simulink model "main"  (R2022a)
settings: Solver=FixedStepDiscrete  StartTime=0.0  StopTime=Inf  FixedStep=(50e-6)-(sim_en*4.995e-5)  RelTol=1e-3  EnableMultiTasking=on
model workspace (MAT data in the model file):
  Param : Simulink.Parameter (value not decoded)
  ac_ok : Simulink.Signal (value not decoded)
  ac_ok_120 : Simulink.Signal (value not decoded)
  bulk_voltage : Simulink.Signal (value not decoded)
  burstduty_integ_max : Simulink.Signal (value not decoded)
  burstduty_integ_min : Simulink.Signal (value not decoded)
  burstduty_ki : Simulink.Signal (value not decoded)
  burstduty_kp : Simulink.Signal (value not decoded)
  calib_ok : Simulink.Signal (value not decoded)
  can_addr1 : Simulink.Signal (value not decoded)
  can_addr2 : Simulink.Signal (value not decoded)
  can_addr3 : Simulink.Signal (value not decoded)
  can_addr4 : Simulink.Signal (value not decoded)
  can_data_rx : Simulink.Signal (value not decoded)
  can_data_tx : Simulink.Signal (value not decoded)
  can_timeout_120 : Simulink.Signal (value not decoded)
  chksum_scircv : Simulink.Signal (value not decoded)
  clllc_en_120 : Simulink.Signal (value not decoded)
  clllc_fault_120 : Simulink.Signal (value not decoded)
  clllc_ok_120 : Simulink.Signal (value not decoded)
  cmpss1h : Simulink.Signal (value not decoded)
  cmpss1l : Simulink.Signal (value not decoded)
  cmpss2h : Simulink.Signal (value not decoded)
  cmpss2l : Simulink.Signal (value not decoded)
  cmpss3h : Simulink.Signal (value not decoded)
  cmpss3l : Simulink.Signal (value not decoded)
  cmpss4h : Simulink.Signal (value not decoded)
  cmpss4l : Simulink.Signal (value not decoded)
  cmpss5h : Simulink.Signal (value not decoded)
  cmpss5l : Simulink.Signal (value not decoded)
  cmpss6h : Simulink.Signal (value not decoded)
  cmpss6l : Simulink.Signal (value not decoded)
  cmpss7h : Simulink.Signal (value not decoded)
  cmpss7l : Simulink.Signal (value not decoded)
  cmpss8h : Simulink.Signal (value not decoded)
  cmpss8l : Simulink.Signal (value not decoded)
  cnt_idle : Simulink.Signal (value not decoded)
  cnt_orps : Simulink.Signal (value not decoded)
  cnt_scircv : Simulink.Signal (value not decoded)
  cnt_scixmt : Simulink.Signal (value not decoded)
  cnt_scixmt_func : Simulink.Signal (value not decoded)
  cnt_temp_mux : Simulink.Signal (value not decoded)
  cnt_vdroop : Simulink.Signal (value not decoded)
  config_ok : Simulink.Signal (value not decoded)
  control_en : Simulink.Signal (value not decoded)
  cp_ready_120 : Simulink.Signal (value not decoded)
  d2d_en : Simulink.Signal (value not decoded)
  dchg_off : Simulink.Signal (value not decoded)
  debug_dacb : Simulink.Signal (value not decoded)
  debug_dacc : Simulink.Signal (value not decoded)
  debug_msg1 : Simulink.Signal (value not decoded)
  debug_msg2 : Simulink.Signal (value not decoded)
  debug_msg3 : Simulink.Signal (value not decoded)
  debug_msg4 : Simulink.Signal (value not decoded)
  debug_msg5 : Simulink.Signal (value not decoded)
  debug_msg6 : Simulink.Signal (value not decoded)
  dir_v2g : Simulink.Signal (value not decoded)
  eoss_llc1 : Simulink.Signal (value not decoded)
  eoss_llc2 : Simulink.Signal (value not decoded)
  eoss_orps : Simulink.Signal (value not decoded)
  fault_ocp : Simulink.Signal (value not decoded)
  fault_otp : Simulink.Signal (value not decoded)
  fault_ovp : Simulink.Signal (value not decoded)
  fut_en : Simulink.Signal (value not decoded)
  fwd_en_120 : Simulink.Signal (value not decoded)
  gain_llc1_sec_idc : Simulink.Signal (value not decoded)
  gain_llc1_temp_sr : Simulink.Signal (value not decoded)
  gain_llc2_sec_idc : Simulink.Signal (value not decoded)
  gain_vbat : Simulink.Signal (value not decoded)
  gain_vbulk : Simulink.Signal (value not decoded)
  gain_vout : Simulink.Signal (value not decoded)
  input_current_phasea : Simulink.Signal (value not decoded)
  input_current_phaseb : Simulink.Signal (value not decoded)
  input_current_phasec : Simulink.Signal (value not decoded)
  input_freq : Simulink.Signal (value not decoded)
  input_power : Simulink.Signal (value not decoded)
  input_voltage_phasea : Simulink.Signal (value not decoded)
  input_voltage_phaseb : Simulink.Signal (value not decoded)
  input_voltage_phasec : Simulink.Signal (value not decoded)
  ishare_arbiter : Simulink.Signal (value not decoded)
  ishare_thresh : Simulink.Signal (value not decoded)
  led_g : Simulink.Signal (value not decoded)
  led_r : Simulink.Signal (value not decoded)
  led_y : Simulink.Signal (value not decoded)
  llc1_burst_integ : Simulink.Signal (value not decoded)
  llc1_burstduty_buffer : Simulink.Signal (value not decoded)
  llc1_pfm_error : Simulink.Signal (value not decoded)
  llc1_pfm_integ : Simulink.Signal (value not decoded)
  llc1_pfm_prop : Simulink.Signal (value not decoded)
  llc1_pri_idc : Simulink.Signal (value not decoded)
  llc1_ps_buffer : Simulink.Signal (value not decoded)
  llc1_pspwm_error : Simulink.Signal (value not decoded)
  llc1_pspwm_integ : Simulink.Signal (value not decoded)
  llc1_pspwm_prop : Simulink.Signal (value not decoded)
  llc1_sec_idc : Simulink.Signal (value not decoded)
  llc1_temp_sr : Simulink.Signal (value not decoded)
  llc1_ts_tbctr_buffer : Simulink.Signal (value not decoded)
  llc2_burst_integ : Simulink.Signal (value not decoded)
  llc2_burstduty_buffer : Simulink.Signal (value not decoded)
  llc2_en : Simulink.Signal (value not decoded)
  llc2_en_buffer : Simulink.Signal (value not decoded)
  llc2_pfm_error : Simulink.Signal (value not decoded)
  llc2_pfm_integ : Simulink.Signal (value not decoded)
  llc2_pfm_prop : Simulink.Signal (value not decoded)
  llc2_pri_idc : Simulink.Signal (value not decoded)
  llc2_ps_buffer : Simulink.Signal (value not decoded)
  llc2_pspwm_error : Simulink.Signal (value not decoded)
  llc2_pspwm_integ : Simulink.Signal (value not decoded)
  llc2_pspwm_prop : Simulink.Signal (value not decoded)
  llc2_sec_idc : Simulink.Signal (value not decoded)
  llc2_temp_sr : Simulink.Signal (value not decoded)
  llc2_ts_tbctr_buffer : Simulink.Signal (value not decoded)
  loop_adcint : Simulink.Signal (value not decoded)
  loop_control : Simulink.Signal (value not decoded)
  loop_idle : Simulink.Signal (value not decoded)
  mid_bulk_voltage : Simulink.Signal (value not decoded)
  mode_120 : Simulink.Signal (value not decoded)
  mode_cc_cv : Simulink.Signal (value not decoded)
  myParam : mpt.Parameter (value not decoded)
  obc_ok_120 : Simulink.Signal (value not decoded)
  offset_llc1_sec_idc : Simulink.Signal (value not decoded)
  offset_llc1_temp_sr : Simulink.Signal (value not decoded)
  offset_llc2_sec_idc : Simulink.Signal (value not decoded)
  offset_vbat : Simulink.Signal (value not decoded)
  offset_vbulk : Simulink.Signal (value not decoded)
  offset_vout : Simulink.Signal (value not decoded)
  openloop_en : Simulink.Signal (value not decoded)
  openloop_fault_en : Simulink.Signal (value not decoded)
  ot_fault_120 : Simulink.Signal (value not decoded)
  pfc_en : Simulink.Signal (value not decoded)
  pfc_en_120 : Simulink.Signal (value not decoded)
  pfc_fw_revision : Simulink.Signal (value not decoded)
  pfc_fw_revision_bootloader : Simulink.Signal (value not decoded)
  pfc_fw_revision_debug : Simulink.Signal (value not decoded)
  pfc_ok : Simulink.Signal (value not decoded)
  pfc_ok_120 : Simulink.Signal (value not decoded)
  pfm_a0 : Simulink.Signal (value not decoded)
  pfm_a1 : Simulink.Signal (value not decoded)
  pfm_integ_max : Simulink.Signal (value not decoded)
  pfm_integ_min : Simulink.Signal (value not decoded)
  pfm_ki : Simulink.Signal (value not decoded)
  pfm_kp : Simulink.Signal (value not decoded)
  pri_fut_en : Simulink.Signal (value not decoded)
  pri_fut_en_buffer : Simulink.Signal (value not decoded)
  pri_halfbridge_en : Simulink.Signal (value not decoded)
  pri_halfbridge_en_buffer : Simulink.Signal (value not decoded)
  pspwm_integ_max : Simulink.Signal (value not decoded)
  pspwm_integ_min : Simulink.Signal (value not decoded)
  pspwm_ki : Simulink.Signal (value not decoded)
  pspwm_kp : Simulink.Signal (value not decoded)
  ref_idclink_max : Simulink.Signal (value not decoded)
  ref_iout : Simulink.Signal (value not decoded)
  ref_iout_calib : Simulink.Signal (value not decoded)
  ref_iout_llc1 : Simulink.Signal (value not decoded)
  ref_iout_llc1_calib : Simulink.Signal (value not decoded)
  ref_iout_llc2 : Simulink.Signal (value not decoded)
  ref_iout_llc2_calib : Simulink.Signal (value not decoded)
  ref_pout : Simulink.Signal (value not decoded)
  ref_ss_llc1 : Simulink.Signal (value not decoded)
  ref_ss_llc2 : Simulink.Signal (value not decoded)
  ref_ss_orps : Simulink.Signal (value not decoded)
  ref_vbat : Simulink.Signal (value not decoded)
  ref_vbat_calib : Simulink.Signal (value not decoded)
  ref_vbulk : Simulink.Signal (value not decoded)
  ref_vbulk_calib : Simulink.Signal (value not decoded)
  ref_vbulk_llc1_calib : Simulink.Signal (value not decoded)
  ref_vbulk_llc2_calib : Simulink.Signal (value not decoded)
  ref_vout : Simulink.Signal (value not decoded)
  ref_vout_calib : Simulink.Signal (value not decoded)
  relay_en : Simulink.Signal (value not decoded)
  reset_flag : Simulink.Signal (value not decoded)
  rev_en_120 : Simulink.Signal (value not decoded)
  runtime_control : Simulink.Signal (value not decoded)
  runtime_idle : Simulink.Signal (value not decoded)
  scircv_buffer : Simulink.Signal (value not decoded)
  scircv_buffer_tmp : Simulink.Signal (value not decoded)
  scircv_buffer_tmp_idx0 : Simulink.Signal (value not decoded)
  scircv_chksum : Simulink.Signal (value not decoded)
  scircv_chksum_ok : Simulink.Signal (value not decoded)
  scircv_parse_ok : Simulink.Signal (value not decoded)
  scixmt_buffer : Simulink.Signal (value not decoded)
  scixmt_chksum : Simulink.Signal (value not decoded)
  scixmt_func : Simulink.Signal (value not decoded)
  scixmt_word0_lsb : Simulink.Signal (value not decoded)
  scixmt_word0_msb : Simulink.Signal (value not decoded)
  scixmt_word1_lsb : Simulink.Signal (value not decoded)
  scixmt_word1_msb : Simulink.Signal (value not decoded)
  scixmt_word2_lsb : Simulink.Signal (value not decoded)
  scixmt_word2_msb : Simulink.Signal (value not decoded)
  scixmt_wr : Simulink.Signal (value not decoded)
  ss_step : Simulink.Signal (value not decoded)
  state_calib : Simulink.Signal (value not decoded)
  state_control : Simulink.Signal (value not decoded)
  state_hkeep : Simulink.Signal (value not decoded)
  status_cmpss : Simulink.Signal (value not decoded)
  status_control : Simulink.Signal (value not decoded)
  status_digin : Simulink.Signal (value not decoded)
  status_digout : Simulink.Signal (value not decoded)
  status_fault : Simulink.Signal (value not decoded)
  status_input : Simulink.Signal (value not decoded)
  status_pfc : Simulink.Signal (value not decoded)
  temp_inlet : Simulink.Signal (value not decoded)
  temp_llc1_fet_hs : Simulink.Signal (value not decoded)
  temp_llc2_fet_hs : Simulink.Signal (value not decoded)
  temp_mux : Simulink.Signal (value not decoded)
  temp_mux_s0 : Simulink.Signal (value not decoded)
  temp_mux_s1 : Simulink.Signal (value not decoded)
  temp_mux_s2 : Simulink.Signal (value not decoded)
  temp_outlet : Simulink.Signal (value not decoded)
  temp_pfc_fet_hsa : Simulink.Signal (value not decoded)
  temp_pfc_fet_hsb : Simulink.Signal (value not decoded)
  temp_pfc_fet_hsc : Simulink.Signal (value not decoded)
  temp_pfc_fet_lsa : Simulink.Signal (value not decoded)
  temp_pfc_fet_lsb : Simulink.Signal (value not decoded)
  temp_pfc_fet_lsc : Simulink.Signal (value not decoded)
  test_mode : Simulink.Signal (value not decoded)
  tfcv_cc : Simulink.Signal (value not decoded)
  tfcv_cc_llc2 : Simulink.Signal (value not decoded)
  tfcv_cv : Simulink.Signal (value not decoded)
  tfcv_sr_en : Simulink.Signal (value not decoded)
  tfv_assert_llc1_pri_idc : Simulink.Signal (value not decoded)
  tfv_assert_llc1_sec_idc : Simulink.Signal (value not decoded)
  tfv_assert_llc1_temp_sr : Simulink.Signal (value not decoded)
  tfv_assert_llc2_pri_idc : Simulink.Signal (value not decoded)
  tfv_assert_llc2_sec_idc : Simulink.Signal (value not decoded)
  tfv_assert_llc2_temp_sr : Simulink.Signal (value not decoded)
  tfv_assert_temp_outlet : Simulink.Signal (value not decoded)
  tfv_assert_vaux_uv : Simulink.Signal (value not decoded)
  tfv_assert_vbat : Simulink.Signal (value not decoded)
  tfv_assert_vbulk : Simulink.Signal (value not decoded)
  tfv_assert_vout : Simulink.Signal (value not decoded)
  tfv_cnt_tz : Simulink.Signal (value not decoded)
  tfv_deassert_llc1_pri_idc : Simulink.Signal (value not decoded)
  tfv_deassert_llc1_sec_idc : Simulink.Signal (value not decoded)
  tfv_deassert_llc1_temp_sr : Simulink.Signal (value not decoded)
  tfv_deassert_llc2_pri_idc : Simulink.Signal (value not decoded)
  tfv_deassert_llc2_sec_idc : Simulink.Signal (value not decoded)
  tfv_deassert_llc2_temp_sr : Simulink.Signal (value not decoded)
  tfv_deassert_temp_outlet : Simulink.Signal (value not decoded)
  tfv_deassert_vaux_uv : Simulink.Signal (value not decoded)
  tfv_deassert_vbat : Simulink.Signal (value not decoded)
  tfv_deassert_vbulk : Simulink.Signal (value not decoded)
  tfv_deassert_vout : Simulink.Signal (value not decoded)
  tfv_llc1_pri_idc : Simulink.Signal (value not decoded)
  tfv_llc1_sec_idc : Simulink.Signal (value not decoded)
  tfv_llc1_temp_sr : Simulink.Signal (value not decoded)
  tfv_llc2_pri_idc : Simulink.Signal (value not decoded)
  tfv_llc2_sec_idc : Simulink.Signal (value not decoded)
  tfv_llc2_temp_sr : Simulink.Signal (value not decoded)
  tfv_temp_outlet : Simulink.Signal (value not decoded)
  tfv_vaux_uv : Simulink.Signal (value not decoded)
  tfv_vbat : Simulink.Signal (value not decoded)
  tfv_vbulk : Simulink.Signal (value not decoded)
  tfv_vout : Simulink.Signal (value not decoded)
  timer_1ms : Simulink.Signal (value not decoded)
  tz : Simulink.Signal (value not decoded)
  valve_en : Simulink.Signal (value not decoded)
  vaux : Simulink.Signal (value not decoded)
  vbat : Simulink.Signal (value not decoded)
  vbulk : Simulink.Signal (value not decoded)
  vout : Simulink.Signal (value not decoded)
undefined symbols (not defined in the file or in its folder): CAN_O_INT, CANA_BASE, Down, GPTRIP1SEL, GPTRIP2SEL, TZ1, TZ2, Up
libraries: hdlsllib x159, simulink x100, c2837xDlib x24, c2807xlib x16, c280xlib x13, c2802xlib x12, canmsglib x8, idelinklib_common x2, c2000lib x1, c281xlib x1
(part 12 of 15)

== system main/Task_Manager/idle/idle_task/status/init/digin//digout_variant_subsystem/sim ==
  sim_digin : Inport
  Data Store Read : DataStoreRead  DataStoreName=dchg_off  IndexOptions=Index vector (dialog)  Indices=1  OutputSizes=1
  Data Store Read1 : DataStoreRead  DataStoreName=temp_mux_s0  IndexOptions=Index vector (dialog)  Indices=1  OutputSizes=1
  Data Store Read2 : DataStoreRead  DataStoreName=pfc_en  IndexOptions=Index vector (dialog)  Indices=1  OutputSizes=1
  Data Store Read3 : DataStoreRead  DataStoreName=temp_mux_s1  IndexOptions=Index vector (dialog)  Indices=1  OutputSizes=1
  Data Store Read4 : DataStoreRead  DataStoreName=temp_mux_s2  IndexOptions=Index vector (dialog)  Indices=1  OutputSizes=1
  Data Store Read5 : DataStoreRead  DataStoreName=valve_en  IndexOptions=Index vector (dialog)  Indices=1  OutputSizes=1
  Data Store Read6 : DataStoreRead  DataStoreName=relay_en  IndexOptions=Index vector (dialog)  Indices=1  OutputSizes=1
  Data Store Read7 : DataStoreRead  DataStoreName=led_r  IndexOptions=Index vector (dialog)  Indices=1  OutputSizes=1
  Data Store Read8 : DataStoreRead  DataStoreName=led_g  IndexOptions=Index vector (dialog)  Indices=1  OutputSizes=1
  Data Store Read9 : DataStoreRead  DataStoreName=led_y  IndexOptions=Index vector (dialog)  Indices=1  OutputSizes=1
  Data Store Write : DataStoreWrite  DataStoreName=ac_ok  IndexOptions=Index vector (dialog)  Indices=1  OutputSizes=1
  Data Store Write1 : DataStoreWrite  DataStoreName=can_addr1  IndexOptions=Index vector (dialog)  Indices=1  OutputSizes=1
  Data Store Write2 : DataStoreWrite  DataStoreName=can_addr2  IndexOptions=Index vector (dialog)  Indices=1  OutputSizes=1
  Data Store Write3 : DataStoreWrite  DataStoreName=can_addr3  IndexOptions=Index vector (dialog)  Indices=1  OutputSizes=1
  Data Store Write4 : DataStoreWrite  DataStoreName=can_addr4  IndexOptions=Index vector (dialog)  Indices=1  OutputSizes=1
  Data Store Write5 : DataStoreWrite  DataStoreName=pfc_ok  IndexOptions=Index vector (dialog)  Indices=1  OutputSizes=1
  Demux : Demux  Outputs=7
  Mux : Mux  Inputs=10
  sim_digout : Outport
  wires:
  sim_digin/1 -> Demux/1
  Demux/6 -> Data Store Write/1
  Demux/7 -> ?
  Demux/1 -> Data Store Write1/1
  Demux/2 -> Data Store Write2/1
  Demux/3 -> Data Store Write3/1
  Demux/4 -> Data Store Write4/1
  Demux/5 -> Data Store Write5/1
  Mux/1 -> sim_digout/1
  Data Store Read7/1 -> Mux/1
  Data Store Read8/1 -> Mux/2
  Data Store Read5/1 -> Mux/9
  Data Store Read4/1 -> Mux/8
  Data Store Read3/1 -> Mux/7
  Data Store Read1/1 -> Mux/6
  Data Store Read/1 -> Mux/4
  Data Store Read2/1 -> Mux/5
  Data Store Read9/1 -> Mux/3
  Data Store Read6/1 -> Mux/10

== system main/Task_Manager/idle/idle_task/status/update_CAN_msg1/OBC_CTRL_MSG_100/G2V_Forward_ON_A2 ==
  Action Port : ActionPort  ActionPortLabel=case [ 162 ]:
  Constant : Constant  Value=0  OutDataTypeStr=boolean  SampleTime=-1
  Constant1 : Constant  OutDataTypeStr=boolean  SampleTime=-1
  Data Store Write1 : DataStoreWrite  DataStoreName=fwd_en_120  IndexOptions=Index vector (dialog)  Indices=1  OutputSizes=1
  Data Store Write16 : DataStoreWrite  DataStoreName=dir_v2g  IndexOptions=Index vector (dialog)  Indices=1  OutputSizes=1
  wires:
  Constant/1 -> Data Store Write16/1
  Constant1/1 -> Data Store Write1/1

== system main/Task_Manager/idle/idle_task/status/update_CAN_msg1/OBC_CTRL_MSG_100/Sleep_A0 ==
  Action Port : ActionPort  ActionPortLabel=case [ 160 ]:
  Constant : Constant  Value=0  OutDataTypeStr=boolean
  Data Store Write16 : DataStoreWrite  DataStoreName=control_en  IndexOptions=Index vector (dialog)  Indices=1  OutputSizes=1
  wires:
  Constant/1 -> Data Store Write16/1

== system main/Task_Manager/idle/idle_task/status/update_CAN_msg1/OBC_CTRL_MSG_100/Stand-by_A1 ==
  Action Port : ActionPort  ActionPortLabel=case [ 161 ]:
  Constant : Constant  OutDataTypeStr=boolean
  Constant2 : Constant  Value=0  OutDataTypeStr=boolean  SampleTime=-1
  Data Store Write1 : DataStoreWrite  DataStoreName=rev_en_120  IndexOptions=Index vector (dialog)  Indices=1  OutputSizes=1
  Data Store Write16 : DataStoreWrite  DataStoreName=control_en  IndexOptions=Index vector (dialog)  Indices=1  OutputSizes=1
  Data Store Write2 : DataStoreWrite  DataStoreName=fwd_en_120  IndexOptions=Index vector (dialog)  Indices=1  OutputSizes=1
  wires:
  Constant/1 -> Data Store Write16/1
  Constant2/1 -> Data Store Write1/1, Data Store Write2/1

== system main/Task_Manager/idle/idle_task/status/update_CAN_msg1/OBC_CTRL_MSG_100/Test_mode_ON_AND_FWD_A4 ==
  Action Port : ActionPort  ActionPortLabel=case [ 164 ]:
  Constant : Constant  OutDataTypeStr=boolean
  Constant1 : Constant  Value=0  OutDataTypeStr=boolean  SampleTime=-1
  Data Store Write1 : DataStoreWrite  DataStoreName=dir_v2g  IndexOptions=Index vector (dialog)  Indices=1  OutputSizes=1
  Data Store Write16 : DataStoreWrite  DataStoreName=test_mode  IndexOptions=Index vector (dialog)  Indices=1  OutputSizes=1
  wires:
  Constant/1 -> Data Store Write16/1
  Constant1/1 -> Data Store Write1/1

== system main/Task_Manager/idle/idle_task/status/update_CAN_msg1/OBC_CTRL_MSG_100/Test_mode_ON_AND_REV_A5 ==
  Action Port : ActionPort  ActionPortLabel=case [ 165 ]:
  Constant : Constant  OutDataTypeStr=boolean
  Constant1 : Constant  OutDataTypeStr=boolean  SampleTime=-1
  Data Store Write1 : DataStoreWrite  DataStoreName=dir_v2g  IndexOptions=Index vector (dialog)  Indices=1  OutputSizes=1
  Data Store Write16 : DataStoreWrite  DataStoreName=test_mode  IndexOptions=Index vector (dialog)  Indices=1  OutputSizes=1
  wires:
  Constant/1 -> Data Store Write16/1
  Constant1/1 -> Data Store Write1/1

== system main/Task_Manager/idle/idle_task/status/update_CAN_msg1/OBC_CTRL_MSG_100/V2G_Reverse_ON_A3 ==
  Action Port : ActionPort  ActionPortLabel=case [ 163 ]:
  Constant : Constant  OutDataTypeStr=boolean
  Constant2 : Constant  OutDataTypeStr=boolean  SampleTime=-1
  Data Store Write16 : DataStoreWrite  DataStoreName=dir_v2g  IndexOptions=Index vector (dialog)  Indices=1  OutputSizes=1
  Data Store Write2 : DataStoreWrite  DataStoreName=rev_en_120  IndexOptions=Index vector (dialog)  Indices=1  OutputSizes=1
  wires:
  Constant/1 -> Data Store Write16/1
  Constant2/1 -> Data Store Write2/1

== system main/Task_Manager/idle/idle_task/status/update_CAN_msg1/OBC_SEC_DATA2_141/Subsystem3 ==
  adc : Inport
  zero_offset : Inport  Port=2
  gain : Inport  Port=3
  Abs : Abs  SaturateOnIntegerOverflow=off
  Product6 : Product  OutDataTypeStr=single
  Saturation1 : Saturate  UpperLimit=4095  LowerLimit=0  OutDataTypeStr=single
  Subtract : Sum  Inputs=+-  AccumDataTypeStr=single  OutDataTypeStr=single
  actual : Outport
  wires:
  Product6/1 -> actual/1
  gain/1 -> Product6/2
  adc/1 -> Subtract/1
  zero_offset/1 -> Subtract/2
  Subtract/1 -> Abs/1
  Saturation1/1 -> Product6/1
  Abs/1 -> Saturation1/1

== system main/Task_Manager/idle/idle_task/status/update_CAN_msg1/OBC_SEC_DATA4_143/Subsystem ==
  Add : Sum  Inputs=++++++++
  Bit Shift1 : hdlsllib/Logic and Bit Operations/Bit Shift  mode=Shift Left Logical  N=1
  Bit Shift2 : hdlsllib/Logic and Bit Operations/Bit Shift  mode=Shift Left Logical  N=2
  Bit Shift3 : hdlsllib/Logic and Bit Operations/Bit Shift  mode=Shift Left Logical  N=3
  Bit Shift4 : hdlsllib/Logic and Bit Operations/Bit Shift  mode=Shift Left Logical  N=5
  Bit Shift5 : hdlsllib/Logic and Bit Operations/Bit Shift  mode=Shift Left Logical  N=6
  Bit Shift6 : hdlsllib/Logic and Bit Operations/Bit Shift  mode=Shift Left Logical  N=4
  Bit Shift7 : hdlsllib/Logic and Bit Operations/Bit Shift  mode=Shift Left Logical  N=7
  Data Store Read10 : DataStoreRead  DataStoreName=dir_v2g  IndexOptions=Index vector (dialog)  Indices=1  OutputSizes=1
  Data Store Read11 : DataStoreRead  DataStoreName=eoss_llc1  IndexOptions=Index vector (dialog)  Indices=1  OutputSizes=1
  Data Store Read12 : DataStoreRead  DataStoreName=calib_ok  IndexOptions=Index vector (dialog)  Indices=1  OutputSizes=1
  Data Store Read13 : DataStoreRead  DataStoreName=openloop_en  IndexOptions=Index vector (dialog)  Indices=1  OutputSizes=1
  Data Store Read14 : DataStoreRead  DataStoreName=fut_en  IndexOptions=Index vector (dialog)  Indices=1  OutputSizes=1
  Data Store Read4 : DataStoreRead  DataStoreName=eoss_llc2  IndexOptions=Index vector (dialog)  Indices=1  OutputSizes=1
  Data Store Read7 : DataStoreRead  DataStoreName=config_ok  IndexOptions=Index vector (dialog)  Indices=1  OutputSizes=1
  Data Store Read9 : DataStoreRead  DataStoreName=control_mode  IndexOptions=Index vector (dialog)  Indices=1  OutputSizes=1
  Data Store Write1 : DataStoreWrite  DataStoreName=sSecCtrlState  IndexOptions=Index vector (dialog)  Indices=1  OutputSizes=1
  Data Store Memory : DataStoreMemory  DataStoreName=control_mode  WriteAfterWriteMsg=warning  ShowAdditionalParam=off
  Data Type Conversion{,1..7,11} (9 alike) : DataTypeConversion  OutDataTypeStr=uint8  SaturateOnIntegerOverflow=off  RndMeth=Floor
  wires:
  Data Store Read11/1 -> Data Type Conversion4/1
  Bit Shift7/1 -> Add/8
  Data Type Conversion7/1 -> Bit Shift7/1
  Data Store Read9/1 -> Data Type Conversion/1
  Data Type Conversion2/1 -> Bit Shift2/1
  Bit Shift1/1 -> Add/2
  Bit Shift5/1 -> Add/7
  Data Store Read14/1 -> Data Type Conversion6/1
  Data Type Conversion5/1 -> Bit Shift4/1
  Bit Shift6/1 -> Add/5
  Data Type Conversion11/1 -> Data Store Write1/1
  Data Store Read13/1 -> Data Type Conversion7/1
  Data Type Conversion4/1 -> Bit Shift6/1
  Data Store Read4/1 -> Data Type Conversion5/1
  Data Store Read10/1 -> Data Type Conversion1/1
  Data Type Conversion/1 -> Add/1
  Bit Shift2/1 -> Add/3
  Bit Shift4/1 -> Add/6
  Add/1 -> Data Type Conversion11/1
  Data Type Conversion1/1 -> Bit Shift1/1
  Data Store Read7/1 -> Data Type Conversion3/1
  Data Store Read12/1 -> Data Type Conversion2/1
  Data Type Conversion6/1 -> Bit Shift5/1
  Data Type Conversion3/1 -> Bit Shift3/1
  Bit Shift3/1 -> Add/4

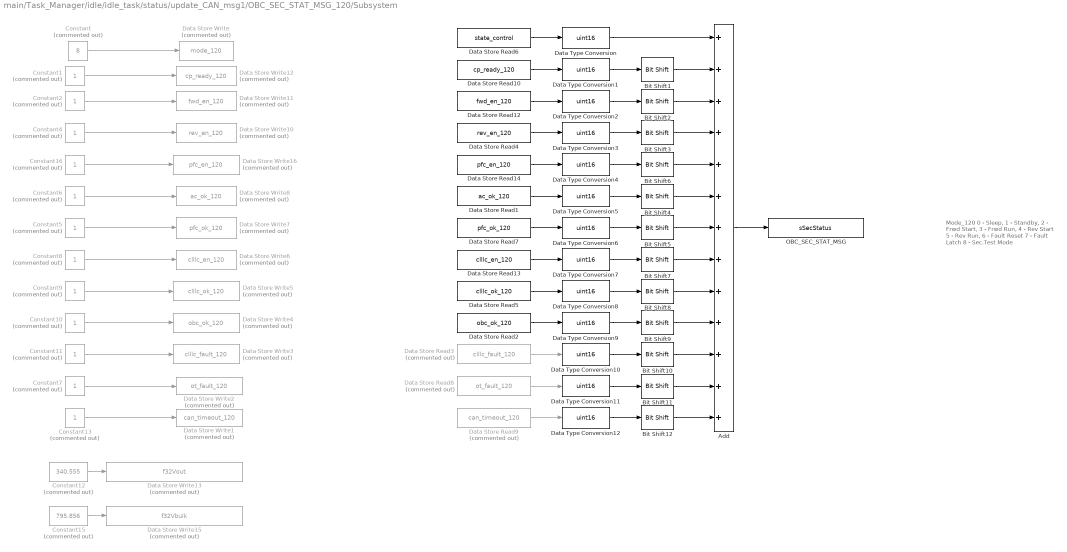
== system main/Task_Manager/idle/idle_task/status/update_CAN_msg1/OBC_SEC_STAT_MSG_120/Subsystem ==
  note: Mode_120
      |
      | 0 - Sleep,
      | 1 - Standby,
      | 2 - Frwd Start,
      | 3 - Frwd Run,
      | 4 - Rev Start
      | 5 - Rev Run,
      | 6 - Fault Reset
      | 7 - Fault Latch
      | 8 - Sec.Test Mode
  Add : Sum  Inputs=+++++++++++++
  Bit Shift1 : hdlsllib/Logic and Bit Operations/Bit Shift  mode=Shift Left Logical  N=4
  Bit Shift10 : hdlsllib/Logic and Bit Operations/Bit Shift  mode=Shift Left Logical  N=13
  Bit Shift11 : hdlsllib/Logic and Bit Operations/Bit Shift  mode=Shift Left Logical  N=14
  Bit Shift12 : hdlsllib/Logic and Bit Operations/Bit Shift  mode=Shift Left Logical  N=15
  Bit Shift2 : hdlsllib/Logic and Bit Operations/Bit Shift  mode=Shift Left Logical  N=5
  Bit Shift3 : hdlsllib/Logic and Bit Operations/Bit Shift  mode=Shift Left Logical  N=6
  Bit Shift4 : hdlsllib/Logic and Bit Operations/Bit Shift  mode=Shift Left Logical  N=8
  Bit Shift5 : hdlsllib/Logic and Bit Operations/Bit Shift  mode=Shift Left Logical  N=9
  Bit Shift6 : hdlsllib/Logic and Bit Operations/Bit Shift  mode=Shift Left Logical  N=7
  Bit Shift7 : hdlsllib/Logic and Bit Operations/Bit Shift  mode=Shift Left Logical  N=10
  Bit Shift8 : hdlsllib/Logic and Bit Operations/Bit Shift  mode=Shift Left Logical  N=11
  Bit Shift9 : hdlsllib/Logic and Bit Operations/Bit Shift  mode=Shift Left Logical  N=12
  Constant : Constant  Commented=on  Value=8  OutDataTypeStr=uint8
  Constant{1..2,4..11,13,16} (12 alike) : Constant  Commented=on  OutDataTypeStr=boolean
  Constant12 : Constant  Commented=on  Value=340.555  OutDataTypeStr=single
  Constant15 : Constant  Commented=on  Value=795.856  OutDataTypeStr=single
  Data Store Read1 : DataStoreRead  DataStoreName=ac_ok_120  IndexOptions=Index vector (dialog)  Indices=1  OutputSizes=1
  Data Store Read10 : DataStoreRead  DataStoreName=cp_ready_120  IndexOptions=Index vector (dialog)  Indices=1  OutputSizes=1
  Data Store Read12 : DataStoreRead  DataStoreName=fwd_en_120  IndexOptions=Index vector (dialog)  Indices=1  OutputSizes=1
  Data Store Read13 : DataStoreRead  DataStoreName=clllc_en_120  IndexOptions=Index vector (dialog)  Indices=1  OutputSizes=1
  Data Store Read14 : DataStoreRead  DataStoreName=pfc_en_120  IndexOptions=Index vector (dialog)  Indices=1  OutputSizes=1
  Data Store Read2 : DataStoreRead  DataStoreName=obc_ok_120  IndexOptions=Index vector (dialog)  Indices=1  OutputSizes=1
  Data Store Read3 : DataStoreRead  Commented=on  DataStoreName=clllc_fault_120  IndexOptions=Index vector (dialog)  Indices=1  OutputSizes=1
  Data Store Read4 : DataStoreRead  DataStoreName=rev_en_120  IndexOptions=Index vector (dialog)  Indices=1  OutputSizes=1
  Data Store Read5 : DataStoreRead  DataStoreName=clllc_ok_120  IndexOptions=Index vector (dialog)  Indices=1  OutputSizes=1
  Data Store Read6 : DataStoreRead  DataStoreName=state_control  IndexOptions=Index vector (dialog)  Indices=1  OutputSizes=1
  Data Store Read7 : DataStoreRead  DataStoreName=pfc_ok_120  IndexOptions=Index vector (dialog)  Indices=1  OutputSizes=1
  Data Store Read8 : DataStoreRead  Commented=on  DataStoreName=ot_fault_120  IndexOptions=Index vector (dialog)  Indices=1  OutputSizes=1
  Data Store Read9 : DataStoreRead  Commented=on  DataStoreName=can_timeout_120  IndexOptions=Index vector (dialog)  Indices=1  OutputSizes=1
  Data Store Write : DataStoreWrite  Commented=on  DataStoreName=mode_120  IndexOptions=Index vector (dialog)  Indices=1  OutputSizes=1
  Data Store Write1 : DataStoreWrite  Commented=on  DataStoreName=can_timeout_120  IndexOptions=Index vector (dialog)  Indices=1  OutputSizes=1
  Data Store Write10 : DataStoreWrite  Commented=on  DataStoreName=rev_en_120  IndexOptions=Index vector (dialog)  Indices=1  OutputSizes=1
  Data Store Write11 : DataStoreWrite  Commented=on  DataStoreName=fwd_en_120  IndexOptions=Index vector (dialog)  Indices=1  OutputSizes=1
  Data Store Write12 : DataStoreWrite  Commented=on  DataStoreName=cp_ready_120  IndexOptions=Index vector (dialog)  Indices=1  OutputSizes=1
  Data Store Write13 : DataStoreWrite  Commented=on  DataStoreName=f32Vout  IndexOptions=Index vector (dialog)  Indices=1  OutputSizes=1
  Data Store Write15 : DataStoreWrite  Commented=on  DataStoreName=f32Vbulk  IndexOptions=Index vector (dialog)  Indices=1  OutputSizes=1
  Data Store Write16 : DataStoreWrite  Commented=on  DataStoreName=pfc_en_120  IndexOptions=Index vector (dialog)  Indices=1  OutputSizes=1
  Data Store Write2 : DataStoreWrite  Commented=on  DataStoreName=ot_fault_120  IndexOptions=Index vector (dialog)  Indices=1  OutputSizes=1
  Data Store Write3 : DataStoreWrite  Commented=on  DataStoreName=clllc_fault_120  IndexOptions=Index vector (dialog)  Indices=1  OutputSizes=1
  Data Store Write4 : DataStoreWrite  Commented=on  DataStoreName=obc_ok_120  IndexOptions=Index vector (dialog)  Indices=1  OutputSizes=1
  Data Store Write5 : DataStoreWrite  Commented=on  DataStoreName=clllc_ok_120  IndexOptions=Index vector (dialog)  Indices=1  OutputSizes=1
  Data Store Write6 : DataStoreWrite  Commented=on  DataStoreName=clllc_en_120  IndexOptions=Index vector (dialog)  Indices=1  OutputSizes=1
  Data Store Write7 : DataStoreWrite  Commented=on  DataStoreName=pfc_ok_120  IndexOptions=Index vector (dialog)  Indices=1  OutputSizes=1
  Data Store Write8 : DataStoreWrite  Commented=on  DataStoreName=ac_ok_120  IndexOptions=Index vector (dialog)  Indices=1  OutputSizes=1
  Data Type Conversion{,1..12} (13 alike) : DataTypeConversion  OutDataTypeStr=uint16  SaturateOnIntegerOverflow=off  RndMeth=Floor
  OBC_SEC_STAT_MSG : DataStoreWrite  DataStoreName=sSecStatus  IndexOptions=Index vector (dialog)  Indices=1  OutputSizes=1
  wires:
  Constant13/1 -> Data Store Write1/1
  Data Store Read12/1 -> Data Type Conversion2/1
  Data Type Conversion1/1 -> Bit Shift1/1
  Bit Shift3/1 -> Add/4
  Bit Shift1/1 -> Add/2
  Data Type Conversion4/1 -> Bit Shift6/1
  Data Type Conversion2/1 -> Bit Shift2/1
  Bit Shift2/1 -> Add/3
  Data Store Read1/1 -> Data Type Conversion5/1
  Bit Shift9/1 -> Add/10
  Data Type Conversion3/1 -> Bit Shift3/1
  Constant2/1 -> Data Store Write11/1
  Data Type Conversion10/1 -> Bit Shift10/1
  Data Store Read8/1 -> Data Type Conversion11/1
  Data Type Conversion7/1 -> Bit Shift7/1
  Data Store Read13/1 -> Data Type Conversion7/1
  Bit Shift8/1 -> Add/9
  Data Type Conversion8/1 -> Bit Shift8/1
  Data Store Read2/1 -> Data Type Conversion9/1
  Data Type Conversion6/1 -> Bit Shift5/1
  Bit Shift6/1 -> Add/5
  Constant5/1 -> Data Store Write7/1
  Constant1/1 -> Data Store Write12/1
  Data Store Read10/1 -> Data Type Conversion1/1
  Data Type Conversion9/1 -> Bit Shift9/1
  Data Type Conversion/1 -> Add/1
  Bit Shift4/1 -> Add/6
  Data Store Read4/1 -> Data Type Conversion3/1
  Bit Shift5/1 -> Add/7
  Constant/1 -> Data Store Write/1
  Data Store Read3/1 -> Data Type Conversion10/1
  Data Type Conversion5/1 -> Bit Shift4/1
  Data Store Read6/1 -> Data Type Conversion/1
  Data Store Read14/1 -> Data Type Conversion4/1
  Constant9/1 -> Data Store Write5/1
  Bit Shift11/1 -> Add/12
  Data Store Read5/1 -> Data Type Conversion8/1
  Bit Shift10/1 -> Add/11
  Data Store Read7/1 -> Data Type Conversion6/1
  Bit Shift7/1 -> Add/8
  Constant11/1 -> Data Store Write3/1
  Constant12/1 -> Data Store Write13/1
  Constant15/1 -> Data Store Write15/1
  Data Type Conversion12/1 -> Bit Shift12/1
  Bit Shift12/1 -> Add/13
  Add/1 -> OBC_SEC_STAT_MSG/1
  Constant8/1 -> Data Store Write6/1
  Constant7/1 -> Data Store Write2/1
  Constant10/1 -> Data Store Write4/1
  Data Type Conversion11/1 -> Bit Shift11/1
  Constant6/1 -> Data Store Write8/1
  Constant4/1 -> Data Store Write10/1
  Constant16/1 -> Data Store Write16/1
  Data Store Read9/1 -> Data Type Conversion12/1

== system main/Task_Manager/idle/idle_task/status/update_CAN_msg1/OBC_SEC_STAT_MSG_120/Subsystem3 ==
  adc : Inport
  zero_offset : Inport  Port=2
  gain : Inport  Port=3
  Abs : Abs  SaturateOnIntegerOverflow=off
  Product6 : Product  OutDataTypeStr=single
  Saturation1 : Saturate  UpperLimit=4095  LowerLimit=0  OutDataTypeStr=single
  Subtract : Sum  Inputs=+-  AccumDataTypeStr=single  OutDataTypeStr=single
  actual : Outport
  wires:
  Product6/1 -> actual/1
  gain/1 -> Product6/2
  adc/1 -> Subtract/1
  zero_offset/1 -> Subtract/2
  Subtract/1 -> Abs/1
  Saturation1/1 -> Product6/1
  Abs/1 -> Saturation1/1

== system main/Task_Manager/init/codegen/init/tztl_clb/clb/System Initialize ==

== system main/Task_Manager/init/codegen/init/tztl_clb/tzctl/System Initialize ==

== system main/Control_State_Machine/Control_Loop/control/configSr/configXbarEpwmtrip/codegen/g2v_prifullbridge/clb/System Outputs1 ==

== system main/Control_State_Machine/Control_Loop/control/configSr/configXbarEpwmtrip/codegen/g2v_prifullbridge/tzctl/System Outputs ==

== system main/Control_State_Machine/Control_Loop/control/configSr/configXbarEpwmtrip/codegen/v2g_prifullbridge/clb/System Outputs3 ==

== system main/Control_State_Machine/Control_Loop/control/configSr/configXbarEpwmtrip/codegen/v2g_prifullbridge/tzctl/System Outputs1 ==

== system main/Task_Manager/Tmr_20mS/codegen/Task_20mS/Rx_Handler/ProcessMB12/Debug_Cmd/Debug En//Dis ==
  Action Port : ActionPort  ActionPortLabel=if(u1 == hex2dec('0xDA'))
  Constant3 : Constant  Value=[2:2]
  Data Store Read1 : DataStoreRead  DataStoreName=u8CanDataRx12  IndexOptions=Index vector (dialog)  Indices=1  OutputSizes=1
  Debug_Dis : Subsystem  TreatAsAtomicUnit=on
  Debug_En : Subsystem  TreatAsAtomicUnit=on
  If : If  IfExpression=u1 == hex2dec('AA')  ElseIfExpressions=u1 ==hex2dec('55')
  Selector3 : Selector  IndexMode=Zero-based  InputPortWidth=8  IndexOptions=Index vector (port)  Indices=[1 3]  OutputSizes=1
  wires:
  Data Store Read1/1 -> Selector3/1
  Constant3/1 -> Selector3/2
  Selector3/1 -> If/1
  If/1 -> Debug_En/Action
  If/2 -> Debug_Dis/Action

== system main/Task_Manager/Tmr_20mS/codegen/Task_20mS/Rx_Handler/ProcessMB12/Debug_Cmd/Open Loop En Dis ==
  Action Port : ActionPort  ActionPortLabel=elseif(u1 == hex2dec('0xDB'))
  Constant3 : Constant  Value=[2:2]
  Data Store Read1 : DataStoreRead  DataStoreName=u8CanDataRx12  IndexOptions=Index vector (dialog)  Indices=1  OutputSizes=1
  Disable Open Loop : Subsystem  TreatAsAtomicUnit=on
  Enable Open Loop : Subsystem  TreatAsAtomicUnit=on
  If : If  IfExpression=u1 == hex2dec('BB')  ElseIfExpressions=u1 ==hex2dec('44')
  Selector3 : Selector  IndexMode=Zero-based  InputPortWidth=8  IndexOptions=Index vector (port)  Indices=[1 3]  OutputSizes=1
  wires:
  Selector3/1 -> If/1
  Constant3/1 -> Selector3/2
  Data Store Read1/1 -> Selector3/1
  If/2 -> Disable Open Loop/Action
  If/1 -> Enable Open Loop/Action

== system main/Task_Manager/Tmr_20mS/codegen/Task_20mS/Rx_Handler/ProcessMB12/Debug_Read/Debug_Cmd ==
  Input : Inport
  Action Port : ActionPort  ActionPortLabel=if(u1 == 1)
  Constant : Constant  OutDataTypeStr=boolean
  Data Store Write1 : DataStoreWrite  DataStoreName=b01_ReadRequest  IndexOptions=Index vector (dialog)  Indices=1  OutputSizes=1
  Data Store Write2 : DataStoreWrite  DataStoreName=u8RdReqMsgPntr  IndexOptions=Index vector (dialog)  Indices=1  OutputSizes=1
  wires:
  Constant/1 -> Data Store Write1/1
  Input/1 -> Data Store Write2/1

== system main/Task_Manager/Tmr_20mS/codegen/Task_20mS/Tx_Handler/Run Tx Routine/TxReadRequest/Tx Cal Data ID145 ==
  Action Port : ActionPort  ActionPortLabel=case [ 208 ]:

== system main/Task_Manager/Tmr_20mS/codegen/Task_20mS/Tx_Handler/Run Tx Routine/TxReadRequest/Tx FW Rev ID144 ==
  Action Port : ActionPort  ActionPortLabel=case [ 240 ]:
  CAN Pack1 : canmsglib/CAN Pack  MsgList=(none)  MsgName=CAN Msg  MsgIDType=Standard (11-bit identifier)  MsgIdentifier=0x144  MsgLength=8  Remote=off  ApplyMinMax=off  BusOutput=off  SignalInfo={}
      settings: SourceProductBaseCode=XP,ME,VN  DataFormat=raw data
  Data Store Read2 : DataStoreRead  DataStoreName=u8FwRevData  IndexOptions=Index vector (dialog)  Indices=1  OutputSizes=1
  eCAN Transmit : c280xlib/eCAN Transmit  chipFamily=C280x  useModule=eCAN_A  mailboxNo=5  messageID=hex2dec('0144')  messageType=Standard (11-bit identifier)  enableBlockingMode=off  postInterrupt=off  interruptLine=0
      settings: SourceProductBaseCode=TIC2000
  wires:
  CAN Pack1/1 -> eCAN Transmit/1
  Data Store Read2/1 -> CAN Pack1/1

== system main/Task_Manager/Tmr_20mS/codegen/Task_20mS/Tx_Handler/Run Tx Routine/TxReadRequest/Tx TxDeb Dat1 146 ==
  Action Port : ActionPort  ActionPortLabel=case [ 209 ]:
  CAN Pack1 : canmsglib/CAN Pack  MsgList=(none)  MsgName=CAN Msg  MsgIDType=Standard (11-bit identifier)  MsgIdentifier=0x146  MsgLength=8  Remote=off  ApplyMinMax=off  BusOutput=off  SignalInfo={}
      settings: SourceProductBaseCode=XP,ME,VN  DataFormat=raw data
  Constant4 : Constant  Value=0  OutDataTypeStr=uint8
  Data Store Read1 : DataStoreRead  DataStoreName=u16Debug0  IndexOptions=Index vector (dialog)  Indices=1  OutputSizes=1
  Data Store Read2 : DataStoreRead  DataStoreName=u16Debug1  IndexOptions=Index vector (dialog)  Indices=1  OutputSizes=1
  Data Store Read3 : DataStoreRead  DataStoreName=u16Debug2  IndexOptions=Index vector (dialog)  Indices=1  OutputSizes=1
  Vector Concatenate : Concatenate  NumInputs=8
  eCAN Transmit : c280xlib/eCAN Transmit  chipFamily=C280x  useModule=eCAN_A  mailboxNo=7  messageID=hex2dec('0146')  messageType=Standard (11-bit identifier)  enableBlockingMode=off  postInterrupt=off  interruptLine=0
      settings: SourceProductBaseCode=TIC2000
  u16 Data to Bytes : Subsystem
  u16 Data to Bytes1 : Subsystem
  u16 Data to Bytes2 : Subsystem
  wires:
  u16 Data to Bytes2/1(u8Lsb) -> Vector Concatenate/3
  u16 Data to Bytes/2(u8Msb) -> Vector Concatenate/2
  Data Store Read2/1 -> u16 Data to Bytes2/1(u16 Data)
  Constant4/1 -> Vector Concatenate/8, Vector Concatenate/7
  Data Store Read3/1 -> u16 Data to Bytes1/1(u16 Data)
  Vector Concatenate/1 -> CAN Pack1/1
  u16 Data to Bytes/1(u8Lsb) -> Vector Concatenate/1
  u16 Data to Bytes1/1(u8Lsb) -> Vector Concatenate/5
  Data Store Read1/1 -> u16 Data to Bytes/1(u16 Data)
  u16 Data to Bytes2/2(u8Msb) -> Vector Concatenate/4
  u16 Data to Bytes1/2(u8Msb) -> Vector Concatenate/6
  CAN Pack1/1 -> eCAN Transmit/1

== system main/Task_Manager/Tmr_20mS/codegen/Task_20mS/Tx_Handler/Run Tx Routine/TxReadRequest/Tx TxDeb Dat2 147 ==
  Action Port : ActionPort  ActionPortLabel=case [ 210 ]:
  CAN Pack1 : canmsglib/CAN Pack  MsgList=(none)  MsgName=CAN Msg  MsgIDType=Standard (11-bit identifier)  MsgIdentifier=0x147  MsgLength=8  Remote=off  ApplyMinMax=off  BusOutput=off  SignalInfo={}
      settings: SourceProductBaseCode=XP,ME,VN  DataFormat=raw data
  Constant4 : Constant  Value=0  OutDataTypeStr=uint8
  Data Store Read1 : DataStoreRead  DataStoreName=u16Debug3  IndexOptions=Index vector (dialog)  Indices=1  OutputSizes=1
  Data Store Read2 : DataStoreRead  DataStoreName=u16Debug4  IndexOptions=Index vector (dialog)  Indices=1  OutputSizes=1
  Data Store Read3 : DataStoreRead  DataStoreName=u16Debug5  IndexOptions=Index vector (dialog)  Indices=1  OutputSizes=1
  Vector Concatenate : Concatenate  NumInputs=8
  eCAN Transmit : c280xlib/eCAN Transmit  chipFamily=C280x  useModule=eCAN_A  mailboxNo=8  messageID=hex2dec('0147')  messageType=Standard (11-bit identifier)  enableBlockingMode=off  postInterrupt=off  interruptLine=0
      settings: SourceProductBaseCode=TIC2000
  u16 Data to Bytes : Subsystem
  u16 Data to Bytes1 : Subsystem
  u16 Data to Bytes2 : Subsystem
  wires:
  u16 Data to Bytes1/2(u8Msb) -> Vector Concatenate/6
  u16 Data to Bytes2/2(u8Msb) -> Vector Concatenate/4
  u16 Data to Bytes1/1(u8Lsb) -> Vector Concatenate/5
  Data Store Read1/1 -> u16 Data to Bytes/1(u16 Data)
  Data Store Read3/1 -> u16 Data to Bytes1/1(u16 Data)
  Vector Concatenate/1 -> CAN Pack1/1
  u16 Data to Bytes/1(u8Lsb) -> Vector Concatenate/1
  CAN Pack1/1 -> eCAN Transmit/1
  Data Store Read2/1 -> u16 Data to Bytes2/1(u16 Data)
  u16 Data to Bytes/2(u8Msb) -> Vector Concatenate/2
  Constant4/1 -> Vector Concatenate/8, Vector Concatenate/7
  u16 Data to Bytes2/1(u8Lsb) -> Vector Concatenate/3

== system main/Task_Manager/Tmr_20mS/codegen/Task_20mS/Tx_Handler/Run Tx Routine/TxStatusData/Tx Sec Status ID120 ==
  Action Port : ActionPort  ActionPortLabel=case [ 0 ]:
  CAN Pack1 : canmsglib/CAN Pack  MsgList=(none)  MsgName=CAN Msg  MsgIDType=Standard (11-bit identifier)  MsgIdentifier=0x120  MsgLength=8  Remote=off  ApplyMinMax=off  BusOutput=off  SignalInfo={}
      settings: SourceProductBaseCode=XP,ME,VN  DataFormat=raw data
  Constant1 : Constant  Value=0.1  OutDataTypeStr=single
  Constant3 : Constant  Value=0.01  OutDataTypeStr=single
  Constant4 : Constant  Value=0.1  OutDataTypeStr=single
  Data Store Read1 : DataStoreRead  DataStoreName=sSecStatus  IndexOptions=Index vector (dialog)  Indices=1  OutputSizes=1
  Data Store Read2 : DataStoreRead  DataStoreName=f32Vout  IndexOptions=Index vector (dialog)  Indices=1  OutputSizes=1
  Data Store Read3 : DataStoreRead  DataStoreName=b00_DebugEnabled  IndexOptions=Index vector (dialog)  Indices=1  OutputSizes=1
  Data Store Read4 : DataStoreRead  DataStoreName=f32Iout  IndexOptions=Index vector (dialog)  Indices=1  OutputSizes=1
  Data Store Read5 : DataStoreRead  DataStoreName=f32Vbulk  IndexOptions=Index vector (dialog)  Indices=1  OutputSizes=1
  Float Data to Bytes : Subsystem
  Float Data to Bytes1 : Subsystem
  Float Data to Bytes2 : Subsystem
  If1 : If  IfExpression=u1 == 1
  TxReadRequest : Subsystem  TreatAsAtomicUnit=on
  Vector Concatenate : Concatenate  NumInputs=8
  eCAN Transmit : c280xlib/eCAN Transmit  chipFamily=C280x  useModule=eCAN_A  mailboxNo=0  messageID=hex2dec('0120')  messageType=Standard (11-bit identifier)  enableBlockingMode=off  postInterrupt=off  interruptLine=0
      settings: SourceProductBaseCode=TIC2000
  u16 Data to Bytes : Subsystem
  wires:
  CAN Pack1/1 -> eCAN Transmit/1
  Data Store Read3/1 -> If1/1
  If1/1 -> TxReadRequest/Action
  Data Store Read1/1 -> u16 Data to Bytes/1(u16 Data)
  u16 Data to Bytes/1(u8Lsb) -> Vector Concatenate/1
  u16 Data to Bytes/2(u8Msb) -> Vector Concatenate/2
  Vector Concatenate/1 -> CAN Pack1/1
  Constant1/1 -> Float Data to Bytes/2(Resol.)
  Data Store Read2/1 -> Float Data to Bytes/1(Float Data)
  Float Data to Bytes/1(u8Lsb) -> Vector Concatenate/3
  Float Data to Bytes/2(u8Msb) -> Vector Concatenate/4
  Data Store Read4/1 -> Float Data to Bytes1/1(Float Data)
  Constant3/1 -> Float Data to Bytes1/2(Resol.)
  Constant4/1 -> Float Data to Bytes2/2(Resol.)
  Data Store Read5/1 -> Float Data to Bytes2/1(Float Data)
  Float Data to Bytes1/1(u8Lsb) -> Vector Concatenate/5
  Float Data to Bytes1/2(u8Msb) -> Vector Concatenate/6
  Float Data to Bytes2/1(u8Lsb) -> Vector Concatenate/7
  Float Data to Bytes2/2(u8Msb) -> Vector Concatenate/8

== system main/Task_Manager/Tmr_20mS/codegen/Task_20mS/Tx_Handler/Run Tx Routine/TxStatusData/Tx Sec1 ID140 ==
  Action Port : ActionPort  ActionPortLabel=case [ 1 ]:
  CAN Pack1 : canmsglib/CAN Pack  MsgList=(none)  MsgName=CAN Msg  MsgIDType=Standard (11-bit identifier)  MsgIdentifier=0x140  MsgLength=8  Remote=off  ApplyMinMax=off  BusOutput=off  SignalInfo={}
      settings: SourceProductBaseCode=XP,ME,VN  DataFormat=raw data
  Constant1 : Constant  Value=2  OutDataTypeStr=uint8
  Constant4 : Constant  Value=0.01  OutDataTypeStr=single
  Data Store Read1 : DataStoreRead  DataStoreName=sSecFault  IndexOptions=Index vector (dialog)  Indices=1  OutputSizes=1
  Data Store Read2 : DataStoreRead  DataStoreName=u16Reserved1  IndexOptions=Index vector (dialog)  Indices=1  OutputSizes=1
  Data Store Read3 : DataStoreRead  DataStoreName=u16Reserved2  IndexOptions=Index vector (dialog)  Indices=1  OutputSizes=1
  Data Store Read5 : DataStoreRead  DataStoreName=f32PriCurrRev  IndexOptions=Index vector (dialog)  Indices=1  OutputSizes=1
  Data Store Write1 : DataStoreWrite  DataStoreName=u8CanTxIndex  IndexOptions=Index vector (dialog)  Indices=1  OutputSizes=1
  Float Data to Bytes2 : Subsystem
  Vector Concatenate : Concatenate  NumInputs=8
  eCAN Transmit : c280xlib/eCAN Transmit  chipFamily=C280x  useModule=eCAN_A  mailboxNo=1  messageID=hex2dec('0140')  messageType=Standard (11-bit identifier)  enableBlockingMode=off  postInterrupt=off  interruptLine=0
      settings: SourceProductBaseCode=TIC2000
  u16 Data to Bytes : Subsystem
  u16 Data to Bytes1 : Subsystem
  u16 Data to Bytes2 : Subsystem
  wires:
  Constant1/1 -> Data Store Write1/1
  Data Store Read2/1 -> u16 Data to Bytes2/1(u16 Data)
  CAN Pack1/1 -> eCAN Transmit/1
  u16 Data to Bytes2/1(u8Lsb) -> Vector Concatenate/3
  u16 Data to Bytes/1(u8Lsb) -> Vector Concatenate/1
  u16 Data to Bytes/2(u8Msb) -> Vector Concatenate/2
  Float Data to Bytes2/2(u8Msb) -> Vector Concatenate/8
  Constant4/1 -> Float Data to Bytes2/2(Resol.)
  Float Data to Bytes2/1(u8Lsb) -> Vector Concatenate/7
  Data Store Read5/1 -> Float Data to Bytes2/1(Float Data)
  u16 Data to Bytes2/2(u8Msb) -> Vector Concatenate/4
  Data Store Read1/1 -> u16 Data to Bytes/1(u16 Data)
  u16 Data to Bytes1/1(u8Lsb) -> Vector Concatenate/5
  Vector Concatenate/1 -> CAN Pack1/1
  u16 Data to Bytes1/2(u8Msb) -> Vector Concatenate/6
  Data Store Read3/1 -> u16 Data to Bytes1/1(u16 Data)

== system main/Task_Manager/Tmr_20mS/codegen/Task_20mS/Tx_Handler/Run Tx Routine/TxStatusData/Tx Sec2 ID141 ==
  Action Port : ActionPort  ActionPortLabel=case [ 2 ]:
  CAN Pack1 : canmsglib/CAN Pack  MsgList=(none)  MsgName=CAN Msg  MsgIDType=Standard (11-bit identifier)  MsgIdentifier=0x141  MsgLength=8  Remote=off  ApplyMinMax=off  BusOutput=off  SignalInfo={}
      settings: SourceProductBaseCode=XP,ME,VN  DataFormat=raw data
  Constant1 : Constant  Value=3  OutDataTypeStr=uint8
  Constant{2..5} (4 alike) : Constant  Value=0.01  OutDataTypeStr=single
  Data Store Read1 : DataStoreRead  DataStoreName=f32Iout1  IndexOptions=Index vector (dialog)  Indices=1  OutputSizes=1
  Data Store Read2 : DataStoreRead  DataStoreName=f32Iout2  IndexOptions=Index vector (dialog)  Indices=1  OutputSizes=1
  Data Store Read4 : DataStoreRead  DataStoreName=f32PriCurrRev1  IndexOptions=Index vector (dialog)  Indices=1  OutputSizes=1
  Data Store Read5 : DataStoreRead  DataStoreName=f32PriCurrRev2  IndexOptions=Index vector (dialog)  Indices=1  OutputSizes=1
  Data Store Write1 : DataStoreWrite  DataStoreName=u8CanTxIndex  IndexOptions=Index vector (dialog)  Indices=1  OutputSizes=1
  Float Data to Bytes : Subsystem
  Float Data to Bytes1 : Subsystem
  Float Data to Bytes2 : Subsystem
  Float Data to Bytes3 : Subsystem
  Vector Concatenate : Concatenate  NumInputs=8
  eCAN Transmit : c280xlib/eCAN Transmit  chipFamily=C280x  useModule=eCAN_A  mailboxNo=2  messageID=hex2dec('0141')  messageType=Standard (11-bit identifier)  enableBlockingMode=off  postInterrupt=off  interruptLine=0
      settings: SourceProductBaseCode=TIC2000
  wires:
  Constant1/1 -> Data Store Write1/1
  Data Store Read4/1 -> Float Data to Bytes1/1(Float Data)
  Data Store Read2/1 -> Float Data to Bytes/1(Float Data)
  Constant2/1 -> Float Data to Bytes/2(Resol.)
  CAN Pack1/1 -> eCAN Transmit/1
  Float Data to Bytes/1(u8Lsb) -> Vector Concatenate/3
  Float Data to Bytes3/1(u8Lsb) -> Vector Concatenate/1
  Float Data to Bytes3/2(u8Msb) -> Vector Concatenate/2
  Float Data to Bytes2/2(u8Msb) -> Vector Concatenate/8
  Constant4/1 -> Float Data to Bytes2/2(Resol.)
  Float Data to Bytes2/1(u8Lsb) -> Vector Concatenate/7
  Data Store Read5/1 -> Float Data to Bytes2/1(Float Data)
  Float Data to Bytes/2(u8Msb) -> Vector Concatenate/4
  Data Store Read1/1 -> Float Data to Bytes3/1(Float Data)
  Float Data to Bytes1/1(u8Lsb) -> Vector Concatenate/5
  Vector Concatenate/1 -> CAN Pack1/1
  Constant3/1 -> Float Data to Bytes1/2(Resol.)
  Float Data to Bytes1/2(u8Msb) -> Vector Concatenate/6
  Constant5/1 -> Float Data to Bytes3/2(Resol.)
